simulink library "lib_lowphy"  (R2023b)
settings: Solver=VariableStepAuto  StartTime=0.0  StopTime=10.0  RelTol=1e-3
undefined symbols (not defined in the file or in its folder): AdvDSPBChannelOutDisplay, AdvDSPBDMemDisplay, AdvDSPBInDisplay, AdvDSPBOutDisplay, dpoly, dspba, dspba_ChannelInVis, dspba_ChannelOutVis, dspba_internal_get_channel_ports, evalAionMaskParam, fft_tb_in, ifft_tb_in, latency, latencyCorrection, max_FFTStages, max_NSubcarriers, primtype, UseDontCare, value
libraries: DSPBAPrim x637, DSPBAControl x55, $bdroot x16, DSPBAModelBus x12, DSPBAUtilities x6, DSPBABase x5, DSPBAWaveformSynth x4, DspbAdvFftLibrary x3, DSPBAVectorUtil x2, DspbAdvVfftPrefix x1
(part 4 of 9)

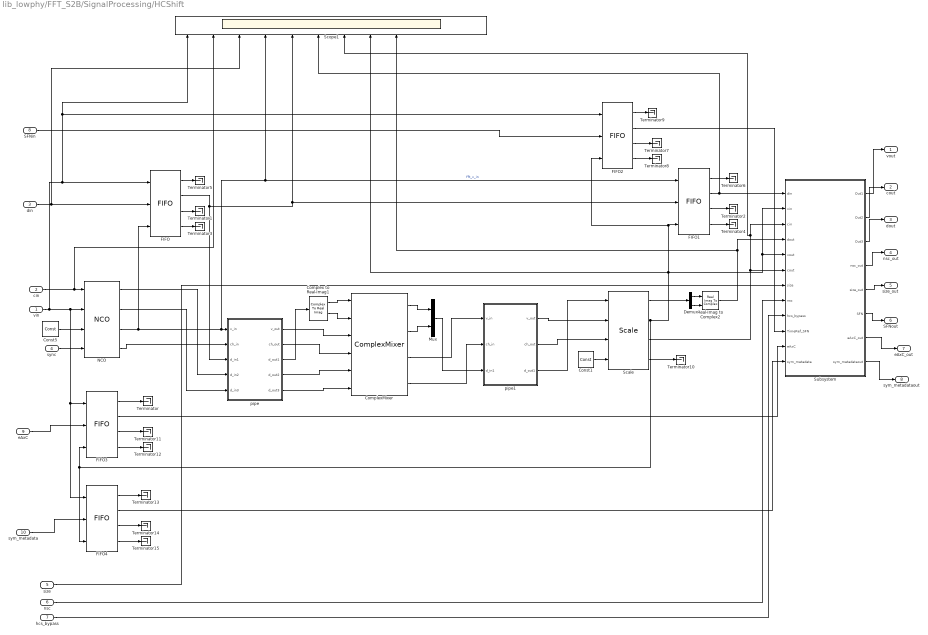
== system lib_lowphy/FFT_S2B/SignalProcessing/HCShift ==
  vin : Inport
  cin : Inport  Port=2
  din : Inport  Port=3
  sync : Inport  Port=4
  size : Inport  Port=5
  nsc : Inport  Port=6
  hcs_bypass : Inport  Port=7
  SFNin : Inport  Port=8
  eAxC : Inport  Port=9
  sym_metadata : Inport  Port=10
  Complex to Real-Imag1 : ComplexToRealImag
  ComplexMixer : DSPBAWaveformSynth/ComplexMixer  nInputRate=dspb_fft_multichannel.ClockRate  nchan=1  nfreq=1  latency=5  simulationMode=Use Global Value  version=20090407
  Const1 : DSPBAPrim/Const  primtype=const  nInputs=0  nOutputs=1  omode=Inherit via internal rule  otype=sfix(16)  scale=2^-15  rndmethod=Unbiased  factor=1  satmethod=Symmetric  shift_vec=[0 1 2 -1]  value=0  inPortNames=['+'; '+';]  outPortNames=[' ']  dspbaimage=dspba_prim.svg  text=fprintf('%s', num2str(value));  style=Optimised  visibilities=8 + 1024  floatPrecision=float32_m23  warnSaturation=on  version=20211007  SampleTime=inf
  Const5 : DSPBAPrim/Const  primtype=const  nInputs=0  nOutputs=1  omode=Specify via dialog  otype=uint(30)  scale=2^0  rndmethod=Unbiased  factor=1  satmethod=Symmetric  shift_vec=[0 1 2 -1]  value=0  inPortNames=['+'; '+';]  outPortNames=[' ']  dspbaimage=dspba_prim.svg  text=fprintf('%s', num2str(value));  style=Optimised  visibilities=8 + 1024  floatPrecision=float32_m23  warnSaturation=on  version=20211007  SampleTime=inf
  Demux : Demux  Outputs=2
  FIFO{,1,3..4} (4 alike) : DSPBAPrim/FIFO  primtype=fifo  nInputs=3  nOutputs=4  omode=Inherit via internal rule  otype=sfix(16)  scale=2^-15  rndmethod=Unbiased  factor=1  satmethod=Symmetric  shift_vec=[0 1 2 -1]  value=[32 4 16]  inPortNames=['w'; 'd'; 'r'; 'f']  outPortNames=['v'; 'q'; 't'; 'f']  dspbaimage=dspba_prim_tall.svg  text=fprintf('fifo');  style=Optimised  visibilities=263168  version=20211007  user_sclr=off
  FIFO2 : DSPBAPrim/FIFO  primtype=fifo  nInputs=3  nOutputs=4  omode=Inherit via internal rule  otype=sfix(16)  scale=2^-15  rndmethod=Unbiased  factor=1  satmethod=Symmetric  shift_vec=[0 1 2 -1]  value=[64 4 16]  inPortNames=['w'; 'd'; 'r'; 'f']  outPortNames=['v'; 'q'; 't'; 'f']  dspbaimage=dspba_prim_tall.svg  text=fprintf('fifo');  style=Optimised  visibilities=263168  version=20211007  user_sclr=off
  Mux : Mux  Inputs=2
  NCO : DSPBAWaveformSynth/NCO  outputRate=dspb_fft_multichannel.ClockRate  otype=sfix(18)  scale=2^-17  accumBitWidth=30  phaseIncrAndInv=7.5e3*2^30/7.68e6  phaseIncrAndInvMap=NCO_addr_offset  rwmode=Read/Write  exposebus=off  version=20090407  SampleTime=-1  expSFDR=108.36  accumPrecision=+/- 0.22888  phaseIncrInMHz=[0.48]  outWidth=3  tableSize=8  latency=17
  Real-Imag to Complex2 : RealImagToComplex
  Scale : DSPBABase/Scale  otype=sfix(16)  scale=2^-15  rndmethod=Biased  factor=1  satmethod=Symmetric  shift_vec=0  latency=3  simulationMode=Use Global Value  version=20130807
  Scope1 : Scope  NumInputPorts=12
  Subsystem : Subsystem
  Terminator{,1..15} (16 alike) : Terminator
  pipe : Subsystem
  pipe1 : Subsystem
  vout : Outport
  cout : Outport  Port=2
  dout : Outport  Port=3
  nsc_out : Outport  Port=4
  size_out : Outport  Port=5
  SFNout : Outport  Port=6
  eAxC_out : Outport  Port=7
  sym_metadataout : Outport  Port=8
  wires:
  NCO/3 -> FIFO/3, FIFO1/1, Scope1/4, pipe/1(v_in)  "fft_v_in"
  Const5/1 -> NCO/3
  cin/1 -> Scope1/2, NCO/1
  vin/1 -> FIFO2/1, Scope1/1, FIFO/1, FIFO4/1, FIFO3/1, NCO/2
  Subsystem/1(Out1) -> vout/1
  Subsystem/2(Out2) -> cout/1
  Subsystem/3(Out3) -> dout/1
  FIFO/3 -> Terminator1/1
  FIFO/4 -> Terminator3/1
  nsc/1 -> Subsystem/8(nsc)
  size/1 -> Subsystem/7(size)
  Subsystem/5(size_out) -> size_out/1
  Subsystem/4(nsc_out) -> nsc_out/1
  hcs_bypass/1 -> Subsystem/9(hcs_bypass)
  sync/1 -> NCO/4
  Real-Imag to Complex2/1 -> Scope1/9, Subsystem/4(dout)
  Scale/2 -> FIFO4/3, FIFO3/3, Scope1/8, Subsystem/2(vin), Subsystem/5(vout), FIFO2/3, FIFO1/3
  Scale/3 -> Scope1/7, Subsystem/3(cin), Subsystem/6(cout)
  FIFO/2 -> FIFO1/2, Scope1/5, pipe/3(d_in1)
  NCO/1 -> pipe/4(d_in2)
  pipe1/1(v_out) -> Scale/2
  NCO/4 -> pipe/2(ch_in)
  Complex to Real-Imag1/2 -> ComplexMixer/2
  pipe1/2(ch_out) -> Scale/3
  pipe/3(d_out1) -> Complex to Real-Imag1/1
  pipe/1(v_out) -> ComplexMixer/3
  Demux/1 -> Real-Imag to Complex2/1
  pipe1/3(d_out1) -> Scale/1
  ComplexMixer/4 -> pipe1/2(ch_in)
  pipe/5(d_out3) -> ComplexMixer/6
  Scale/4 -> Terminator10/1
  pipe/4(d_out2) -> ComplexMixer/5
  Const1/1 -> Scale/4
  ComplexMixer/1 -> Mux/1
  Scale/1 -> Demux/1
  Complex to Real-Imag1/1 -> ComplexMixer/1
  Demux/2 -> Real-Imag to Complex2/2
  pipe/2(ch_out) -> ComplexMixer/4
  ComplexMixer/3 -> pipe1/1(v_in)
  Mux/1 -> pipe1/3(d_in1)
  ComplexMixer/2 -> Mux/2
  NCO/2 -> pipe/5(d_in3)
  FIFO1/2 -> Scope1/6, Subsystem/1(din)
  FIFO1/4 -> Terminator4/1
  FIFO1/3 -> Terminator2/1
  FIFO/1 -> Terminator5/1
  FIFO1/1 -> Terminator6/1
  din/1 -> Scope1/3, FIFO/2
  SFNin/1 -> FIFO2/2
  FIFO2/3 -> Terminator7/1
  FIFO2/4 -> Terminator8/1
  FIFO2/1 -> Terminator9/1
  FIFO2/2 -> Subsystem/10(TimeRef_SFN)
  Subsystem/6(SFN) -> SFNout/1
  eAxC/1 -> FIFO3/2
  sym_metadata/1 -> FIFO4/2
  FIFO3/1 -> Terminator/1
  FIFO3/3 -> Terminator11/1
  FIFO3/4 -> Terminator12/1
  FIFO4/1 -> Terminator13/1
  FIFO4/3 -> Terminator14/1
  FIFO4/4 -> Terminator15/1
  Subsystem/7(eAxC_out) -> eAxC_out/1
  Subsystem/8(sym_metadataout) -> sym_metadataout/1
  FIFO3/2 -> Subsystem/11(eAxC)
  FIFO4/2 -> Subsystem/12(sym_metadata)

== system lib_lowphy/FFT_S2B/SignalProcessing/RXGainComp ==
  vin : Inport
  chin : Inport  Port=2
  din : Inport  Port=3
  nsc : Inport  Port=4
  size : Inport  Port=5
  fft_gain_re : Inport  Port=6
  fft_gain_im : Inport  Port=7
  time_in : Inport  Port=8
  eAxC : Inport  Port=9
  sym_metadata : Inport  Port=10
  Mult : DSPBAPrim/Mult  primtype=mult  nInputs=2  nOutputs=1  omode=Inherit via internal rule  otype=sfix(16)  scale=2^-15  rndmethod=Unbiased  factor=1  satmethod=Symmetric  shift_vec=[0 1 2 -1]  value=0  inPortNames=[' '; ' ';]  outPortNames=[' ']  dspbaimage=dspba_prim.svg  text=fprintf('X');  style=Optimised  visibilities=8+2^18+2^19  floatPrecision=float32_m23  floatRounding=correct  advOptions=[]  version=20211007
  Real-Imag to Complex : RealImagToComplex
  Scale1 : DSPBAPrim/Convert  primtype=convert  nInputs=1  nOutputs=1  omode=Specify via dialog  otype=sfix(16)  scale=2^-14  rndmethod=Biased  factor=1  satmethod=Symmetric  shift_vec=[0 1 2 -1]  value=round([0:255]/17)  inPortNames=[' '; ' ';]  outPortNames=[' '; 'c']  dspbaimage=dspba_prim_wide.svg  text=fprintf('convert');  style=Optimised  visibilities=8+64+256+2^17  clipdetect=off  floatPrecision=float32_m23  advOptions=[]  version=20211007
  SynthesisInfo : DSPBAPrim/SynthesisInfo  primtype=synthinfo  nInputs=0  nOutputs=0  omode=Inherit via internal rule  otype=sfix(16)  scale=2^-15  rndmethod=Truncate  factor=1  satmethod=Symmetric  shift_vec=[0 1 2 -1]  value=99  inPortNames=[' '; ' ';]  outPortNames=[' ']  dspbaimage=dspba_prim_ctrl.jpg  text=fprintf('Style=%s', style);  style=Scheduled  visibilities=2^17+2^18+2^19+2^20+2^21+2^22+2^23+2^24  constraintPair=None  constraintRelation=>  constraintLimit=2  modelRefSign=+  modelRef=''  showSchedule=off  simulationMode=Use Global Value  resetMinimization=Conditional - On for ChannelIn/Out only  version=20220106
  channel_RXG1_in : DSPBAPrim/ChannelIn  primtype=channelin  nInputs=dspba_internal_get_channel_ports(gcb)  nOutputs=dspba_internal_get_channel_ports(gcb)  omode=Inherit via internal rule  otype=sfix(16)  scale=2^-15  rndmethod=Unbiased  factor=1  satmethod=Symmetric  shift_vec=[0 1 2 -1]  value=8  inPortNames=['v'; 'c'; '0'; '1'; '2'; '3'; '4'; '5'; '6'; '7'; '8'; '9'; 'A'; 'B'; 'D'; 'E'; 'F'; 'G'; 'H'; 'I'; 'J'; 'K'; 'L'; 'M'; 'N'; 'O'; 'P'; 'Q'; 'R'; 'S'; 'T'; 'U'; 'W'; 'X'; 'Y'; 'Z']  outPortNames=['v'; 'c'; '0'; '1'; '2'; '3'; '4'; '5'; '6'; '7'; '8'; '9'; 'A'; 'B'; 'D'; 'E'; 'F'; 'G'; 'H'; 'I'; 'J'; 'K'; 'L'; 'M'; 'N'; 'O'; 'P'; 'Q'; 'R'; 'S'; 'T'; 'U'; 'W'; 'X'; 'Y'; 'Z']  dspbaimage=dspba_prim_channel_tall.svg  text=fprintf('In');  style=Optimised  dataSignals=8  foldingEnabled=off  channels=1  sampleRate=200  packetBeginPresent=off  packetBeginEnabled=off  visibilities=dspba_ChannelInVis(gcb)  latencyCorrection=0  scheduleOrigin=on  version=20211214
  channel_RXG1_out : DSPBAPrim/ChannelOut  primtype=channelout  nInputs=dspba_internal_get_channel_ports(gcb)  nOutputs=dspba_internal_get_channel_ports(gcb)  omode=Inherit via internal rule  otype=sfix(16)  scale=2^-15  rndmethod=Unbiased  factor=1  satmethod=Symmetric  shift_vec=[0 1 2 -1]  value=6  inPortNames=['v'; 'c'; '0'; '1'; '2'; '3'; '4'; '5'; '6'; '7'; '8'; '9'; 'A'; 'B'; 'D'; 'E'; 'F'; 'G'; 'H'; 'I'; 'J'; 'K'; 'L'; 'M'; 'N'; 'O'; 'P'; 'Q'; 'R'; 'S'; 'T'; 'U'; 'W'; 'X'; 'Y'; 'Z']  outPortNames=['v'; 'c'; '0'; '1'; '2'; '3'; '4'; '5'; '6'; '7'; '8'; '9'; 'A'; 'B'; 'D'; 'E'; 'F'; 'G'; 'H'; 'I'; 'J'; 'K'; 'L'; 'M'; 'N'; 'O'; 'P'; 'Q'; 'R'; 'S'; 'T'; 'U'; 'W'; 'X'; 'Y'; 'Z']  dspbaimage=dspba_prim_channel_tall.svg  text=fprintf('Out%s', AdvDSPBChannelOutDisplay(latency));  style=Optimised  dataSignals=6  foldingEnabled=off  channels=1  sampleRate=200  packetBeginPresent=off  packetBeginEnabled=off  visibilities=dspba_ChannelOutVis(gcb)  latency=8  latencyCorrection=0  version=20211214
  vout : Outport
  chout : Outport  Port=2
  dout : Outport  Port=3
  nsc_out : Outport  Port=4
  size_out : Outport  Port=5
  time_out : Outport  Port=6
  eAxC_out : Outport  Port=7
  sym_metadata_out : Outport  Port=8
  wires:
  Scale1/1 -> channel_RXG1_out/3
  Mult/1 -> Scale1/1
  channel_RXG1_out/1 -> vout/1
  channel_RXG1_out/2 -> chout/1
  channel_RXG1_in/1 -> channel_RXG1_out/1
  channel_RXG1_in/2 -> channel_RXG1_out/2
  channel_RXG1_out/3 -> dout/1
  channel_RXG1_in/3 -> Mult/1
  chin/1 -> channel_RXG1_in/2
  vin/1 -> channel_RXG1_in/1
  din/1 -> channel_RXG1_in/3
  channel_RXG1_out/4 -> size_out/1
  channel_RXG1_out/5 -> nsc_out/1
  channel_RXG1_in/4 -> channel_RXG1_out/4
  channel_RXG1_in/5 -> channel_RXG1_out/5
  size/1 -> channel_RXG1_in/4
  nsc/1 -> channel_RXG1_in/5
  fft_gain_re/1 -> channel_RXG1_in/6
  fft_gain_im/1 -> channel_RXG1_in/7
  channel_RXG1_in/7 -> Real-Imag to Complex/2
  time_in/1 -> channel_RXG1_in/8
  channel_RXG1_in/8 -> channel_RXG1_out/6
  channel_RXG1_out/6 -> time_out/1
  channel_RXG1_in/6 -> Real-Imag to Complex/1
  Real-Imag to Complex/1 -> Mult/2
  eAxC/1 -> channel_RXG1_in/9
  sym_metadata/1 -> channel_RXG1_in/10
  channel_RXG1_out/7 -> eAxC_out/1
  channel_RXG1_out/8 -> sym_metadata_out/1
  channel_RXG1_in/9 -> channel_RXG1_out/7
  channel_RXG1_in/10 -> channel_RXG1_out/8

== system lib_lowphy/FFT_S2B/SignalProcessing/RXScaling ==
  vin : Inport
  chin : Inport  Port=2
  size : Inport  Port=3
  din : Inport  Port=4
  nsc : Inport  Port=5
  fft_shift : Inport  Port=6
  time_in : Inport  Port=7
  eAxC : Inport  Port=8
  sym_metadata : Inport  Port=9
  Complex to Real-Imag : ComplexToRealImag
  Real-Imag to Complex : RealImagToComplex
  Scale1 : DSPBAPrim/Convert  primtype=convert  nInputs=1  nOutputs=1  omode=Specify via dialog  otype=sfix(16)  scale=Rx_scaling  rndmethod=Biased  factor=1  satmethod=Symmetric  shift_vec=[0 1 2 -1]  value=round([0:255]/17)  inPortNames=[' '; ' ';]  outPortNames=[' '; 'c']  dspbaimage=dspba_prim_wide.svg  text=fprintf('convert');  style=Optimised  visibilities=8+64+256+2^17  clipdetect=off  floatPrecision=float32_m23  advOptions=[]  version=20211007
  Scale2 : DSPBAPrim/Convert  primtype=convert  nInputs=1  nOutputs=1  omode=Specify via dialog  otype=sfix(16)  scale=Rx_scaling  rndmethod=Biased  factor=1  satmethod=Symmetric  shift_vec=[0 1 2 -1]  value=round([0:255]/17)  inPortNames=[' '; ' ';]  outPortNames=[' '; 'c']  dspbaimage=dspba_prim_wide.svg  text=fprintf('convert');  style=Optimised  visibilities=8+64+256+2^17  clipdetect=off  floatPrecision=float32_m23  advOptions=[]  version=20211007
  Scope : Scope  NumInputPorts=3
  Shift : DSPBAPrim/Shift  primtype=shift  nInputs=2  nOutputs=1  omode=Inherit via internal rule  otype=sfix(16)  scale=Rx_scaling  rndmethod=Unbiased  factor=1  satmethod=Symmetric  shift_vec=[0 1 2 -1]  value=0  inPortNames=['a'; 'b';]  outPortNames=[' ']  dspbaimage=dspba_prim.svg  text=fprintf('a >> b');  style=Optimised  visibilities=8  version=20211007
  Shift1 : DSPBAPrim/Shift  primtype=shift  nInputs=2  nOutputs=1  omode=Inherit via internal rule  otype=sfix(16)  scale=Rx_scaling  rndmethod=Unbiased  factor=1  satmethod=Symmetric  shift_vec=[0 1 2 -1]  value=0  inPortNames=['a'; 'b';]  outPortNames=[' ']  dspbaimage=dspba_prim.svg  text=fprintf('a >> b');  style=Optimised  visibilities=8  version=20211007
  SynthesisInfo : DSPBAPrim/SynthesisInfo  primtype=synthinfo  nInputs=0  nOutputs=0  omode=Inherit via internal rule  otype=sfix(16)  scale=2^-15  rndmethod=Truncate  factor=1  satmethod=Symmetric  shift_vec=[0 1 2 -1]  value=99  inPortNames=[' '; ' ';]  outPortNames=[' ']  dspbaimage=dspba_prim_ctrl.jpg  text=fprintf('Style=%s', style);  style=Scheduled  visibilities=2^17+2^18+2^19+2^20+2^21+2^22+2^23+2^24  constraintPair=None  constraintRelation=>  constraintLimit=2  modelRefSign=+  modelRef=''  showSchedule=off  simulationMode=Use Global Value  resetMinimization=Conditional - On for ChannelIn/Out only  version=20220106
  channel_RXS1_in : DSPBAPrim/ChannelIn  primtype=channelin  nInputs=dspba_internal_get_channel_ports(gcb)  nOutputs=dspba_internal_get_channel_ports(gcb)  omode=Inherit via internal rule  otype=sfix(16)  scale=2^-15  rndmethod=Unbiased  factor=1  satmethod=Symmetric  shift_vec=[0 1 2 -1]  value=8  inPortNames=['v'; 'c'; '0'; '1'; '2'; '3'; '4'; '5'; '6'; '7'; '8'; '9'; 'A'; 'B'; 'D'; 'E'; 'F'; 'G'; 'H'; 'I'; 'J'; 'K'; 'L'; 'M'; 'N'; 'O'; 'P'; 'Q'; 'R'; 'S'; 'T'; 'U'; 'W'; 'X'; 'Y'; 'Z']  outPortNames=['v'; 'c'; '0'; '1'; '2'; '3'; '4'; '5'; '6'; '7'; '8'; '9'; 'A'; 'B'; 'D'; 'E'; 'F'; 'G'; 'H'; 'I'; 'J'; 'K'; 'L'; 'M'; 'N'; 'O'; 'P'; 'Q'; 'R'; 'S'; 'T'; 'U'; 'W'; 'X'; 'Y'; 'Z']  dspbaimage=dspba_prim_channel_tall.svg  text=fprintf('In');  style=Optimised  dataSignals=8  foldingEnabled=off  channels=1  sampleRate=200  packetBeginPresent=off  packetBeginEnabled=off  visibilities=dspba_ChannelInVis(gcb)  latencyCorrection=0  scheduleOrigin=on  version=20211214
  channel_RXS1_out : DSPBAPrim/ChannelOut  primtype=channelout  nInputs=dspba_internal_get_channel_ports(gcb)  nOutputs=dspba_internal_get_channel_ports(gcb)  omode=Inherit via internal rule  otype=sfix(16)  scale=2^-15  rndmethod=Unbiased  factor=1  satmethod=Symmetric  shift_vec=[0 1 2 -1]  value=7  inPortNames=['v'; 'c'; '0'; '1'; '2'; '3'; '4'; '5'; '6'; '7'; '8'; '9'; 'A'; 'B'; 'D'; 'E'; 'F'; 'G'; 'H'; 'I'; 'J'; 'K'; 'L'; 'M'; 'N'; 'O'; 'P'; 'Q'; 'R'; 'S'; 'T'; 'U'; 'W'; 'X'; 'Y'; 'Z']  outPortNames=['v'; 'c'; '0'; '1'; '2'; '3'; '4'; '5'; '6'; '7'; '8'; '9'; 'A'; 'B'; 'D'; 'E'; 'F'; 'G'; 'H'; 'I'; 'J'; 'K'; 'L'; 'M'; 'N'; 'O'; 'P'; 'Q'; 'R'; 'S'; 'T'; 'U'; 'W'; 'X'; 'Y'; 'Z']  dspbaimage=dspba_prim_channel_tall.svg  text=fprintf('Out%s', AdvDSPBChannelOutDisplay(latency));  style=Optimised  dataSignals=7  foldingEnabled=off  channels=1  sampleRate=200  packetBeginPresent=off  packetBeginEnabled=off  visibilities=dspba_ChannelOutVis(gcb)  latency=6  latencyCorrection=0  version=20211214
  vout : Outport
  chout : Outport  Port=2
  dout : Outport  Port=3
  size_out : Outport  Port=4
  nsc_out : Outport  Port=5
  time_out : Outport  Port=6
  eAxCout : Outport  Port=7
  sym_metadataout : Outport  Port=8
  wires:
  channel_RXS1_out/7 -> time_out/1
  channel_RXS1_out/6 -> nsc_out/1
  channel_RXS1_out/2 -> chout/1
  Scale1/1 -> channel_RXS1_out/3
  Shift/1 -> Scale1/1
  channel_RXS1_in/8 -> channel_RXS1_out/7
  channel_RXS1_in/7 -> Shift/2, Shift1/2
  channel_RXS1_in/6 -> channel_RXS1_out/6
  channel_RXS1_in/5 -> channel_RXS1_out/5
  channel_RXS1_out/1 -> vout/1
  nsc/1 -> channel_RXS1_in/6
  din/1 -> Complex to Real-Imag/1
  size/1 -> channel_RXS1_in/5
  channel_RXS1_out/5 -> size_out/1
  vin/1 -> channel_RXS1_in/1
  channel_RXS1_in/2 -> channel_RXS1_out/2
  Complex to Real-Imag/1 -> channel_RXS1_in/3
  fft_shift/1 -> channel_RXS1_in/7
  chin/1 -> channel_RXS1_in/2
  time_in/1 -> channel_RXS1_in/8
  Complex to Real-Imag/2 -> channel_RXS1_in/4
  channel_RXS1_in/1 -> channel_RXS1_out/1
  Real-Imag to Complex/1 -> dout/1
  channel_RXS1_out/4 -> Real-Imag to Complex/2
  channel_RXS1_out/3 -> Real-Imag to Complex/1
  Shift1/1 -> Scale2/1
  channel_RXS1_in/3 -> Scope/1, Shift/1, Scope/2
  Scale2/1 -> channel_RXS1_out/4
  channel_RXS1_in/4 -> Shift1/1
  eAxC/1 -> channel_RXS1_in/9
  sym_metadata/1 -> channel_RXS1_in/10
  channel_RXS1_out/8 -> eAxCout/1
  channel_RXS1_out/9 -> sym_metadataout/1
  channel_RXS1_in/9 -> channel_RXS1_out/8
  channel_RXS1_in/10 -> channel_RXS1_out/9

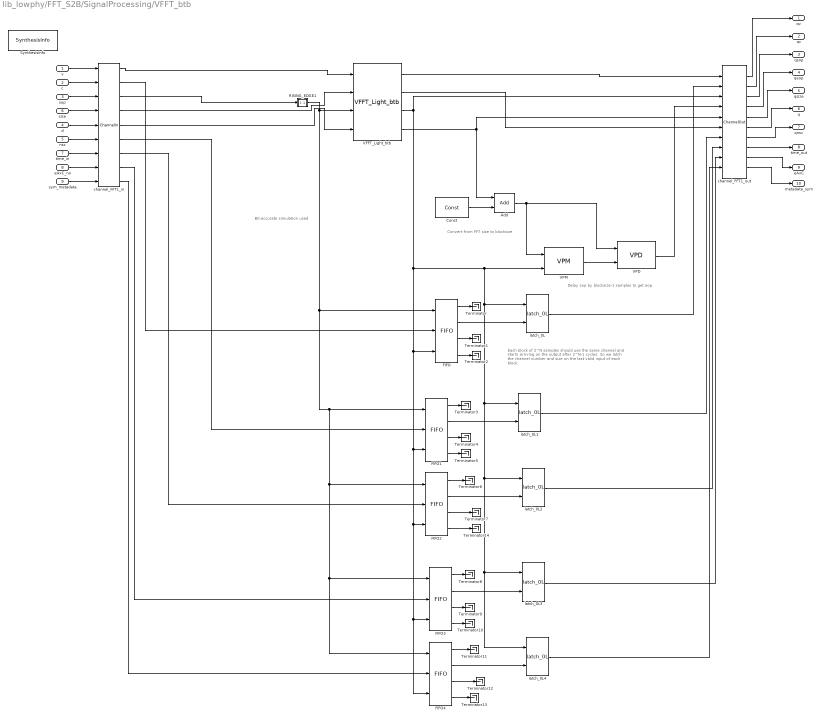
== system lib_lowphy/FFT_S2B/SignalProcessing/VFFT_btb ==
  note: Bit-accurate simulation used
  note: Each block of 2^N samples should use the same channel
      | and starts arriving on the output after 2^N-1 cycles.
      |
      | So we latch the channel number and size on
      |  the last valid input of each block.
  note: Convert from FFT size to blocksize
  note: Delay sop by blocksize-1 samples to get eop.
  v : Inport
  c : Inport  Port=2
  sop : Inport  Port=3
  d : Inport  Port=4
  nsc : Inport  Port=5
  size : Inport  Port=6
  time_in : Inport  Port=7
  eAxC_no : Inport  Port=8
  sym_metadata : Inport  Port=9
  Add : DSPBAPrim/Add  primtype=add  nInputs=evalAionMaskParam(gcb,'value',1)  nOutputs=1  omode=Specify via dialog  otype=fixdt(0,adderWidth,0)  scale=0  rndmethod=Unbiased  factor=1  satmethod=Symmetric  shift_vec=[0 1 2 -1]  value=2  inPortNames=[' '; ' ';]  outPortNames=[' ']  dspbaimage=dspba_prim.svg  text=fprintf('+');  style=Optimised  visibilities=1032+2^17+2^18+2^19  genFPC=off  floatRounding=correct  advOptions=[]  version=20211007
  Const : DSPBAPrim/Const  primtype=const  nInputs=0  nOutputs=1  omode=Inherit via internal rule  otype=sfix(16)  scale=2^-15  rndmethod=Unbiased  factor=1  satmethod=Symmetric  shift_vec=[0 1 2 -1]  value=subchannelbits  inPortNames=['+'; '+';]  outPortNames=[' ']  dspbaimage=dspba_prim.svg  text=fprintf('%s', num2str(value));  style=Optimised  visibilities=8 + 1024  floatPrecision=float32_m23  warnSaturation=on  version=20211007  SampleTime=inf
  FIFO{,1..4} (5 alike) : DSPBAPrim/FIFO  primtype=fifo  nInputs=3  nOutputs=4  omode=Inherit via internal rule  otype=sfix(16)  scale=2^-15  rndmethod=Unbiased  factor=1  satmethod=Symmetric  shift_vec=[0 1 2 -1]  value=[2^(maxSize-minSize) 4 16]  inPortNames=['w'; 'd'; 'r'; 'f']  outPortNames=['v'; 'q'; 't'; 'f']  dspbaimage=dspba_prim_tall.svg  text=fprintf('fifo');  style=Optimised  visibilities=263168  version=20211007  user_sclr=off
  RISING_EDGE1 : Subsystem
  SynthesisInfo : DSPBAPrim/SynthesisInfo  primtype=synthinfo  nInputs=0  nOutputs=0  omode=Inherit via internal rule  otype=sfix(16)  scale=2^-15  rndmethod=Truncate  factor=1  satmethod=Symmetric  shift_vec=[0 1 2 -1]  value=99  inPortNames=[' '; ' ';]  outPortNames=[' ']  dspbaimage=dspba_prim_ctrl.jpg  text=fprintf('Style=%s', style);  style=Scheduled  visibilities=2^17+2^18+2^19+2^20+2^21+2^22+2^23+2^24  constraintPair=None  constraintRelation=>  constraintLimit=2  modelRefSign=+  modelRef=''  showSchedule=off  simulationMode=Bit Accurate  resetMinimization=Conditional - On for ChannelIn/Out only  version=20220106
  Terminator{,1..14} (15 alike) : Terminator
  VFFT_Light_btb : DspbAdvVfftPrefix/VFFT_Light_btb  IFFT=IFFT  subchannels=subchannels  br_in=br_in  maxSize=maxSize  minSize=minSize  in_type=in_type  type_strings=type_strings  faithful=faithful  wirecount=1
  VPD : DspbAdvFftLibrary/Private/VPD  N=maxBlocksizeBits
  VPM : DspbAdvFftLibrary/Private/VPM  N=maxBlocksizeBits
  channel_FFT1_in : DSPBAPrim/ChannelIn  primtype=channelin  nInputs=dspba_internal_get_channel_ports(gcb)  nOutputs=dspba_internal_get_channel_ports(gcb)  omode=Inherit via internal rule  otype=sfix(16)  scale=2^-15  rndmethod=Unbiased  factor=1  satmethod=Symmetric  shift_vec=[0 1 2 -1]  value=7  inPortNames=['v'; 'c'; '0'; '1'; '2'; '3'; '4'; '5'; '6'; '7'; '8'; '9'; 'a'; 'b']  outPortNames=['v'; 'c'; '0'; '1'; '2'; '3'; '4'; '5'; '6'; '7'; '8'; '9'; 'a'; 'b']  dspbaimage=dspba_prim_channel_tall.svg  text=fprintf('In');  style=Optimised  dataSignals=7  foldingEnabled=off  channels=1  sampleRate=200  packetBeginPresent=off  packetBeginEnabled=off  visibilities=dspba_ChannelInVis(gcb)  latencyCorrection=0  scheduleOrigin=on  version=20211214
  channel_FFT1_out : DSPBAPrim/ChannelOut  primtype=channelout  nInputs=dspba_internal_get_channel_ports(gcb)  nOutputs=dspba_internal_get_channel_ports(gcb)  omode=Inherit via internal rule  otype=sfix(16)  scale=2^-15  rndmethod=Unbiased  factor=1  satmethod=Symmetric  shift_vec=[0 1 2 -1]  value=8  inPortNames=['v'; 'c'; '0'; '1'; '2'; '3'; '4'; '5'; '6'; '7'; '8'; '9']  outPortNames=['v'; 'c'; '0'; '1'; '2'; '3'; '4'; '5'; '6'; '7'; '8'; '9']  dspbaimage=dspba_prim_channel_tall.svg  text=fprintf('Out');  style=Optimised  dataSignals=8  foldingEnabled=off  channels=1  sampleRate=200  packetBeginPresent=off  packetBeginEnabled=off  visibilities=dspba_ChannelOutVis(gcb)  latency=75  latencyCorrection=0  version=20211214
  latch_0L{,1..4} (5 alike) : DSPBAControl/latch_0L
  qv : Outport
  qc : Outport  Port=2
  qsop : Outport  Port=3
  qeop : Outport  Port=4
  qsize : Outport  Port=5
  q : Outport  Port=6
  qnsc : Outport  Port=7
  time_out : Outport  Port=8
  eAxC : Outport  Port=9
  metadata_sym : Outport  Port=10
  wires:
  v/1 -> channel_FFT1_in/1
  c/1 -> channel_FFT1_in/2
  channel_FFT1_out/1 -> qv/1
  channel_FFT1_out/2 -> qc/1
  VFFT_Light_btb/1 -> channel_FFT1_out/1
  sop/1 -> channel_FFT1_in/3
  channel_FFT1_out/3 -> qsop/1
  size/1 -> channel_FFT1_in/4
  d/1 -> channel_FFT1_in/5
  channel_FFT1_in/1 -> VFFT_Light_btb/1
  channel_FFT1_in/2 -> FIFO/2
  RISING_EDGE1/1(q) -> FIFO/1, FIFO4/1, FIFO3/1, FIFO2/1, FIFO1/1, VFFT_Light_btb/3
  FIFO/2 -> latch_0L/2
  latch_0L/1 -> channel_FFT1_out/2
  FIFO/1 -> Terminator/1
  FIFO/3 -> Terminator1/1
  FIFO/4 -> Terminator2/1
  channel_FFT1_in/4 -> VFFT_Light_btb/2
  channel_FFT1_in/5 -> VFFT_Light_btb/4
  VPM/1 -> VPD/2
  channel_FFT1_out/6 -> q/1
  channel_FFT1_out/5 -> qsize/1
  channel_FFT1_out/4 -> qeop/1
  VFFT_Light_btb/2 -> channel_FFT1_out/6
  VPD/1 -> channel_FFT1_out/4
  VFFT_Light_btb/4 -> Add/1, channel_FFT1_out/5
  Add/1 -> VPD/1, VPM/1
  Const/1 -> Add/2
  nsc/1 -> channel_FFT1_in/6
  latch_0L1/1 -> channel_FFT1_out/7
  channel_FFT1_out/7 -> qnsc/1
  FIFO1/4 -> Terminator5/1
  FIFO1/3 -> Terminator4/1
  FIFO1/1 -> Terminator3/1
  FIFO1/2 -> latch_0L1/2
  channel_FFT1_in/6 -> FIFO1/2
  channel_FFT1_in/3 -> RISING_EDGE1/1(d)
  time_in/1 -> channel_FFT1_in/7
  channel_FFT1_out/8 -> time_out/1
  VFFT_Light_btb/3 -> channel_FFT1_out/3, FIFO4/3, FIFO3/3, FIFO2/3, FIFO1/3, FIFO/3, latch_0L4/1, latch_0L3/1, latch_0L2/1, latch_0L1/1, latch_0L/1, VPM/2
  FIFO2/1 -> Terminator6/1
  FIFO2/2 -> latch_0L2/2
  latch_0L2/1 -> channel_FFT1_out/8
  FIFO2/3 -> Terminator7/1
  channel_FFT1_in/7 -> FIFO2/2
  eAxC_no/1 -> channel_FFT1_in/8
  sym_metadata/1 -> channel_FFT1_in/9
  FIFO3/4 -> Terminator10/1
  FIFO3/1 -> Terminator8/1
  FIFO3/2 -> latch_0L3/2
  FIFO4/2 -> latch_0L4/2
  FIFO4/3 -> Terminator12/1
  FIFO3/3 -> Terminator9/1
  FIFO4/1 -> Terminator11/1
  FIFO4/4 -> Terminator13/1
  channel_FFT1_out/9 -> eAxC/1
  channel_FFT1_out/10 -> metadata_sym/1
  channel_FFT1_in/8 -> FIFO3/2
  channel_FFT1_in/9 -> FIFO4/2
  latch_0L3/1 -> channel_FFT1_out/9
  latch_0L4/1 -> channel_FFT1_out/10
  FIFO2/4 -> Terminator14/1

== system lib_lowphy/PhaseCompensation/PhasorGenerate/ChangeDetection ==
  In1 : Inport
  CmpNE : DSPBAPrim/CmpNE  primtype=cmpne  nInputs=2  nOutputs=1  omode=boolean  otype=sfix(16)  scale=2^-15  rndmethod=Unbiased  factor=1  satmethod=Symmetric  shift_vec=[0 1 2 -1]  value=0  inPortNames=[' '; ' ';]  outPortNames=[' ']  dspbaimage=dspba_prim.svg  text=fprintf('~=');  style=Optimised  visibilities=0  advOptions=[]  version=20211007
  SampleDelay : DSPBAPrim/SampleDelay  primtype=sampdelay  nInputs=1  nOutputs=1  omode=Inherit via internal rule  otype=sfix(16)  scale=2^-15  rndmethod=Unbiased  factor=1  satmethod=Symmetric  shift_vec=[0 1 2 -1]  floatPrecision=float32_m23  value=1  inPortNames=[' '; ' ';]  outPortNames=[' ']  dspbaimage=dspba_prim.svg  text=dpoly(1, eye(1,value+1), 'z')  style=Optimised  visibilities=8 + 1024 + 2^17 + 2^18  flexible=off  slackgroup=0  augmented=0  version=20211007  advOptions=[]
  Out1 : Outport
  wires:
  In1/1 -> CmpNE/1, SampleDelay/1
  SampleDelay/1 -> CmpNE/2
  CmpNE/1 -> Out1/1

== system lib_lowphy/PhaseCompensation_lite/SOP_EOP_gen/Rising_edge ==
  in : Inport
  Const : DSPBAPrim/Const  primtype=const  nInputs=0  nOutputs=1  omode=Specify via dialog  otype=ufix(1)  scale=0  rndmethod=Unbiased  factor=1  satmethod=Symmetric  shift_vec=[0 1 2 -1]  value=1  inPortNames=['+'; '+';]  outPortNames=[' ']  dspbaimage=dspba_prim.svg  text=fprintf('%s', num2str(value));  style=Optimised  visibilities=8 + 1024 + 2^18 + 2^20  floatPrecision=float32_m23  warnSaturation=on  version=20211007  SampleTime=inf
  Convert : DSPBAPrim/Convert  primtype=convert  nInputs=1  nOutputs=1  omode=Specify via dialog  otype=ufix(1)  scale=0  rndmethod=Unbiased  factor=1  satmethod=None  shift_vec=[0 1 2 -1]  value=round([0:255]/17)  inPortNames=[' '; ' ';]  outPortNames=[' '; 'c']  dspbaimage=dspba_prim_wide.svg  text=fprintf('convert');  style=Optimised  visibilities=8+64+256+2^17  clipdetect=off  floatPrecision=float32_m23  advOptions=[]  version=20211007
  Finite State Machine : DSPBAUtilities/Finite State Machine  desc_file=fsm_control_rising_edge.fsm  latency=0  simulationMode=Bit And Cycle Accurate  finiteStateMachine=on
  GPIn : DSPBAPrim/GPIn  Commented=through  primtype=gpin  nInputs=evalAionMaskParam(gcb,'value',1)  nOutputs=evalAionMaskParam(gcb,'value',1)  omode=Inherit via internal rule  otype=sfix(16)  scale=2^-15  rndmethod=Unbiased  factor=1  satmethod=Symmetric  shift_vec=[0 1 2 -1]  value=1  inPortNames=[' ' ' ' ' ' ' ' ' ' ' ' ' ' ' ' ' ' ' ' ' ' ' ' ' ' ' ' ' ' ' ' ' ' ' ' ' ' ' ' ' ' ' ' ' ' ' ' ' ' ' ' ' ' ' ' ' ' ' ' ' ' ' ' ' ' ' ' ' ']'  outPortNames=[' ' ' ' ' ' ' ' ' ' ' ' ' ' ' ' ' ' ' ' ' ' ' ' ' ' ' ' ' ' ' ' ' ' ' ' ' ' ' ' ' ' ' ' ' ' ' ' ' ' ' ' ' ' ' ' ' ' ' ' ' ' ' ' ' ' ' ' ' ']'  dspbaimage=dspba_prim_channel_tall.svg  text=fprintf('GPIn%s', AdvDSPBInDisplay(latencyCorrection));  style=Optimised  visibilities=1024  latencyCorrection=0  scheduleOrigin=on  version=20211214
  GPOut : DSPBAPrim/GPOut  Commented=through  primtype=gpout  nInputs=evalAionMaskParam(gcb,'value',1)  nOutputs=evalAionMaskParam(gcb,'value',1)  omode=Inherit via internal rule  otype=sfix(16)  scale=2^-15  rndmethod=Unbiased  factor=1  satmethod=Symmetric  shift_vec=[0 1 2 -1]  value=1  inPortNames=[' ' ' ' ' ' ' ' ' ' ' ' ' ' ' ' ' ' ' ' ' ' ' ' ' ' ' ' ' ' ' ' ' ' ' ' ' ' ' ' ' ' ' ' ' ' ' ' ' ' ' ' ' ' ' ' ' ' ' ' ' ' ' ' ' ' ' ' ' ']'  outPortNames=[' ' ' ' ' ' ' ' ' ' ' ' ' ' ' ' ' ' ' ' ' ' ' ' ' ' ' ' ' ' ' ' ' ' ' ' ' ' ' ' ' ' ' ' ' ' ' ' ' ' ' ' ' ' ' ' ' ' ' ' ' ' ' ' ' ' ' ' ' ']'  dspbaimage=dspba_prim_channel_tall.svg  text=fprintf('GPOut%s', AdvDSPBOutDisplay(latency, latencyCorrection));  style=Optimised  visibilities=1024  latency=0  latencyCorrection=0  version=20211214
  SynthesisInfo : DSPBAPrim/SynthesisInfo  Commented=on  primtype=synthinfo  nInputs=0  nOutputs=0  omode=Inherit via internal rule  otype=sfix(16)  scale=2^-15  rndmethod=Truncate  factor=1  satmethod=Symmetric  shift_vec=[0 1 2 -1]  value=99  inPortNames=[' '; ' ';]  outPortNames=[' ']  dspbaimage=dspba_prim_ctrl.jpg  text=fprintf('Style=%s', style);  style=Scheduled  visibilities=2^17+2^18+2^19+2^20+2^21+2^22+2^23+2^24  constraintPair=GPIn to GPOut  constraintRelation==  constraintLimit=0  modelRefSign=+  modelRef=''  showSchedule=off  simulationMode=Use Global Value  resetMinimization=Conditional - On for ChannelIn/Out only  version=20220106
  rising_edge : Outport
  wires:
  Convert/1 -> Finite State Machine/2
  in/1 -> GPIn/1
  GPOut/1 -> rising_edge/1
  Const/1 -> Finite State Machine/1
  Finite State Machine/1 -> GPOut/1
  GPIn/1 -> Convert/1

== system lib_lowphy/PhaseCompensation_lite/SOP_EOP_gen/falling_edge ==
  in : Inport
  Const : DSPBAPrim/Const  primtype=const  nInputs=0  nOutputs=1  omode=Specify via dialog  otype=ufix(1)  scale=0  rndmethod=Unbiased  factor=1  satmethod=Symmetric  shift_vec=[0 1 2 -1]  value=1  inPortNames=['+'; '+';]  outPortNames=[' ']  dspbaimage=dspba_prim.svg  text=fprintf('%s', num2str(value));  style=Optimised  visibilities=8 + 1024 + 2^18 + 2^20  floatPrecision=float32_m23  warnSaturation=on  version=20211007  SampleTime=inf
  Convert : DSPBAPrim/Convert  primtype=convert  nInputs=1  nOutputs=1  omode=Specify via dialog  otype=ufix(1)  scale=0  rndmethod=Unbiased  factor=1  satmethod=None  shift_vec=[0 1 2 -1]  value=round([0:255]/17)  inPortNames=[' '; ' ';]  outPortNames=[' '; 'c']  dspbaimage=dspba_prim_wide.svg  text=fprintf('convert');  style=Optimised  visibilities=8+64+256+2^17  clipdetect=off  floatPrecision=float32_m23  advOptions=[]  version=20211007
  Finite State Machine : DSPBAUtilities/Finite State Machine  desc_file=fsm_control_falling_edge.fsm  latency=0  simulationMode=Bit And Cycle Accurate  finiteStateMachine=on
  GPIn : DSPBAPrim/GPIn  Commented=through  primtype=gpin  nInputs=evalAionMaskParam(gcb,'value',1)  nOutputs=evalAionMaskParam(gcb,'value',1)  omode=Inherit via internal rule  otype=sfix(16)  scale=2^-15  rndmethod=Unbiased  factor=1  satmethod=Symmetric  shift_vec=[0 1 2 -1]  value=1  inPortNames=[' ' ' ' ' ' ' ' ' ' ' ' ' ' ' ' ' ' ' ' ' ' ' ' ' ' ' ' ' ' ' ' ' ' ' ' ' ' ' ' ' ' ' ' ' ' ' ' ' ' ' ' ' ' ' ' ' ' ' ' ' ' ' ' ' ' ' ' ' ']'  outPortNames=[' ' ' ' ' ' ' ' ' ' ' ' ' ' ' ' ' ' ' ' ' ' ' ' ' ' ' ' ' ' ' ' ' ' ' ' ' ' ' ' ' ' ' ' ' ' ' ' ' ' ' ' ' ' ' ' ' ' ' ' ' ' ' ' ' ' ' ' ' ']'  dspbaimage=dspba_prim_channel_tall.svg  text=fprintf('GPIn%s', AdvDSPBInDisplay(latencyCorrection));  style=Optimised  visibilities=1024  latencyCorrection=0  scheduleOrigin=on  version=20211214
  GPOut : DSPBAPrim/GPOut  Commented=through  primtype=gpout  nInputs=evalAionMaskParam(gcb,'value',1)  nOutputs=evalAionMaskParam(gcb,'value',1)  omode=Inherit via internal rule  otype=sfix(16)  scale=2^-15  rndmethod=Unbiased  factor=1  satmethod=Symmetric  shift_vec=[0 1 2 -1]  value=1  inPortNames=[' ' ' ' ' ' ' ' ' ' ' ' ' ' ' ' ' ' ' ' ' ' ' ' ' ' ' ' ' ' ' ' ' ' ' ' ' ' ' ' ' ' ' ' ' ' ' ' ' ' ' ' ' ' ' ' ' ' ' ' ' ' ' ' ' ' ' ' ' ']'  outPortNames=[' ' ' ' ' ' ' ' ' ' ' ' ' ' ' ' ' ' ' ' ' ' ' ' ' ' ' ' ' ' ' ' ' ' ' ' ' ' ' ' ' ' ' ' ' ' ' ' ' ' ' ' ' ' ' ' ' ' ' ' ' ' ' ' ' ' ' ' ' ']'  dspbaimage=dspba_prim_channel_tall.svg  text=fprintf('GPOut%s', AdvDSPBOutDisplay(latency, latencyCorrection));  style=Optimised  visibilities=1024  latency=0  latencyCorrection=0  version=20211214
  SynthesisInfo : DSPBAPrim/SynthesisInfo  Commented=on  primtype=synthinfo  nInputs=0  nOutputs=0  omode=Inherit via internal rule  otype=sfix(16)  scale=2^-15  rndmethod=Truncate  factor=1  satmethod=Symmetric  shift_vec=[0 1 2 -1]  value=99  inPortNames=[' '; ' ';]  outPortNames=[' ']  dspbaimage=dspba_prim_ctrl.jpg  text=fprintf('Style=%s', style);  style=Scheduled  visibilities=2^17+2^18+2^19+2^20+2^21+2^22+2^23+2^24  constraintPair=GPIn to GPOut  constraintRelation==  constraintLimit=0  modelRefSign=+  modelRef=''  showSchedule=off  simulationMode=Use Global Value  resetMinimization=Conditional - On for ChannelIn/Out only  version=20220106
  falling_edge : Outport
  wires:
  Convert/1 -> Finite State Machine/2
  in/1 -> GPIn/1
  GPOut/1 -> falling_edge/1
  Const/1 -> Finite State Machine/1
  Finite State Machine/1 -> GPOut/1
  GPIn/1 -> Convert/1

== system lib_lowphy/iFFT_B2S/B2S/B2S_Inst ==
  vin : Inport
  chin : Inport  Port=2
  din : Inport  Port=3
  FFTSize : Inport  Port=4
  cplen : Inport  Port=5
  nprb : Inport  Port=6
  BitCombine : DSPBAPrim/BitCombine  primtype=bitcombine  nInputs=2  nOutputs=1  omode=Inherit via internal rule  otype=sfix(16)  scale=2^-15  rndmethod=Unbiased  factor=1  satmethod=Symmetric  shift_vec=[0 1 2 -1]  value=0  inPortNames=['l'; 'h';]  outPortNames=[' ']  dspbaimage=dspba_prim.svg  text=fprintf('[h,l]');  style=Optimised  visibilities=8+2  version=20211007
  CB : Subsystem
  GPIn : DSPBAPrim/GPIn  primtype=gpin  nInputs=evalAionMaskParam(gcb,'value',1)  nOutputs=evalAionMaskParam(gcb,'value',1)  omode=Inherit via internal rule  otype=sfix(16)  scale=2^-15  rndmethod=Unbiased  factor=1  satmethod=Symmetric  shift_vec=[0 1 2 -1]  value=6  inPortNames=[' ' ' ' ' ' ' ' ' ' ' ' ' ' ' ' ' ' ' ' ' ' ' ' ' ' ' ' ' ' ' ' ' ' ' ' ' ' ' ' ' ' ' ' ' ' ' ' ' ' ' ' ' ' ' ' ' ' ' ' ' ' ' ' ' ' ' ' ' ']'  outPortNames=[' ' ' ' ' ' ' ' ' ' ' ' ' ' ' ' ' ' ' ' ' ' ' ' ' ' ' ' ' ' ' ' ' ' ' ' ' ' ' ' ' ' ' ' ' ' ' ' ' ' ' ' ' ' ' ' ' ' ' ' ' ' ' ' ' ' ' ' ' ']'  dspbaimage=dspba_prim_channel_tall.svg  text=fprintf('GPIn');  style=Optimised  visibilities=1024  latencyCorrection=0  scheduleOrigin=on  version=20211214
  GPOut : DSPBAPrim/GPOut  primtype=gpout  nInputs=evalAionMaskParam(gcb,'value',1)  nOutputs=evalAionMaskParam(gcb,'value',1)  omode=Inherit via internal rule  otype=sfix(16)  scale=2^-15  rndmethod=Unbiased  factor=1  satmethod=Symmetric  shift_vec=[0 1 2 -1]  value=3  inPortNames=[' ' ' ' ' ' ' ' ' ' ' ' ' ' ' ' ' ' ' ' ' ' ' ' ' ' ' ' ' ' ' ' ' ' ' ' ' ' ' ' ' ' ' ' ' ' ' ' ' ' ' ' ' ' ' ' ' ' ' ' ' ' ' ' ' ' ' ' ' ']'  outPortNames=[' ' ' ' ' ' ' ' ' ' ' ' ' ' ' ' ' ' ' ' ' ' ' ' ' ' ' ' ' ' ' ' ' ' ' ' ' ' ' ' ' ' ' ' ' ' ' ' ' ' ' ' ' ' ' ' ' ' ' ' ' ' ' ' ' ' ' ' ' ']'  dspbaimage=dspba_prim_channel_tall.svg  text=fprintf('GPOut');  style=Optimised  visibilities=1024  latency=8  latencyCorrection=0  version=20211214
  MemandMux : Subsystem
  SynthesisInfo : DSPBAPrim/SynthesisInfo  primtype=synthinfo  nInputs=0  nOutputs=0  omode=Inherit via internal rule  otype=sfix(16)  scale=2^-15  rndmethod=Truncate  factor=1  satmethod=Symmetric  shift_vec=[0 1 2 -1]  value=99  inPortNames=[' '; ' ';]  outPortNames=[' ']  dspbaimage=dspba_prim_ctrl.jpg  text=fprintf('Style=%s', style);  style=Scheduled  visibilities=2^17+2^18+2^19+2^20+2^21+2^22+2^23+2^24  constraintPair=GPIn to GPOut  constraintRelation=>=  constraintLimit=2  modelRefSign=+  modelRef=''  showSchedule=off  simulationMode=Use Global Value  resetMinimization=On - Always (for ChannelIn/Out or GPIn/Out)  version=20220106
  vout : Outport  VectorParamsAs1DForOutWhenUnconnected=off
  cout : Outport  Port=2  VectorParamsAs1DForOutWhenUnconnected=off
  q : Outport  Port=3  VectorParamsAs1DForOutWhenUnconnected=off
  wires:
  GPIn/5 -> CB/4(cplen)
  CB/7(AntNo) -> MemandMux/4(Ant_sel)
  GPIn/1 -> CB/1(vin)
  GPIn/2 -> CB/2(chin)
  GPIn/3 -> MemandMux/5(data_in)  "data_in"
  GPIn/4 -> CB/3(FFTSize)
  CB/5(rba) -> BitCombine/2
  CB/8(rdaddr1) -> BitCombine/1
  CB/2(Wr_Antenna_no) -> MemandMux/2(AntennaCurId)
  CB/3(Wr_ptr) -> MemandMux/3(Wraddr)
  BitCombine/1 -> MemandMux/6(rdaddr)
  MemandMux/1(dout) -> GPOut/1
  MemandMux/3(dv_out) -> GPOut/3
  MemandMux/2(ch_out) -> GPOut/2
  CB/1(rddv) -> MemandMux/7(rd_dv_in)
  CB/6(We) -> MemandMux/1(dv_we)
  vin/1 -> GPIn/1
  chin/1 -> GPIn/2
  din/1 -> GPIn/3  "data_in"
  FFTSize/1 -> GPIn/4
  cplen/1 -> GPIn/5
  GPOut/2 -> cout/1
  GPOut/1 -> q/1
  GPOut/3 -> vout/1
  GPIn/6 -> CB/5(nprb)
  nprb/1 -> GPIn/6

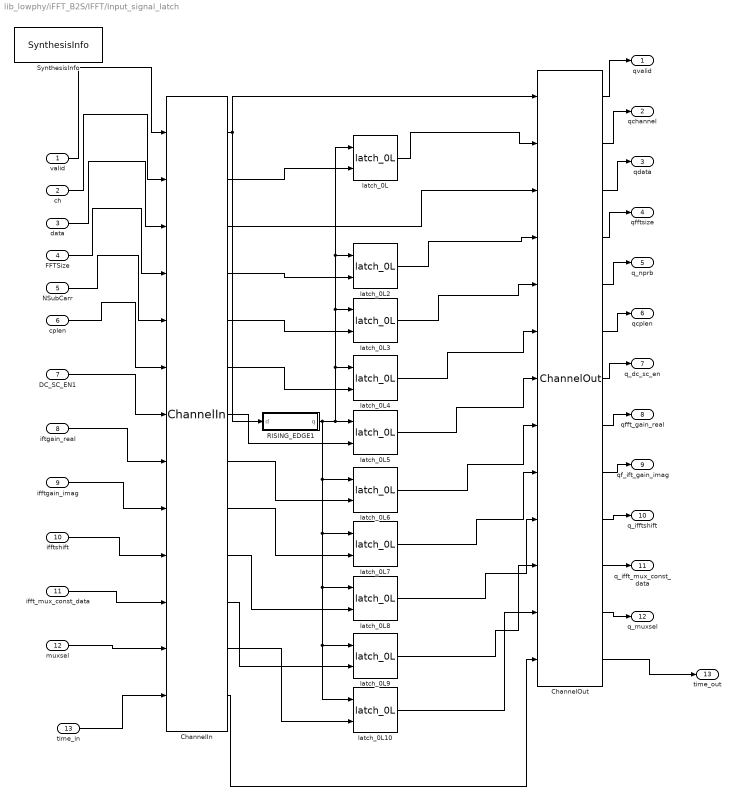
== system lib_lowphy/iFFT_B2S/IFFT/Input_signal_latch ==
  valid : Inport
  ch : Inport  Port=2
  data : Inport  Port=3
  FFTSize : Inport  Port=4
  NSubCarr : Inport  Port=5
  cplen : Inport  Port=6
  DC_SC_EN1 : Inport  Port=7
  iftgain_real : Inport  Port=8
  ifftgain_imag : Inport  Port=9
  ifftshift : Inport  Port=10
  ifft_mux_const_data : Inport  Port=11
  muxsel : Inport  Port=12
  time_in : Inport  Port=13
  ChannelIn : DSPBAPrim/ChannelIn  primtype=channelin  nInputs=dspba_internal_get_channel_ports(gcb)  nOutputs=dspba_internal_get_channel_ports(gcb)  omode=Inherit via internal rule  otype=sfix(16)  scale=2^-15  rndmethod=Unbiased  factor=1  satmethod=Symmetric  shift_vec=[0 1 2 -1]  value=11  inPortNames=['v'; 'c'; '0'; '1'; '2'; '3'; '4'; '5'; '6'; '7'; '8'; '9'; 'A'; 'B'; 'D'; 'E'; 'F'; 'G'; 'H'; 'I'; 'J'; 'K'; 'L'; 'M'; 'N'; 'O'; 'P'; 'Q'; 'R'; 'S'; 'T'; 'U'; 'W'; 'X'; 'Y'; 'Z']  outPortNames=['v'; 'c'; '0'; '1'; '2'; '3'; '4'; '5'; '6'; '7'; '8'; '9'; 'A'; 'B'; 'D'; 'E'; 'F'; 'G'; 'H'; 'I'; 'J'; 'K'; 'L'; 'M'; 'N'; 'O'; 'P'; 'Q'; 'R'; 'S'; 'T'; 'U'; 'W'; 'X'; 'Y'; 'Z']  dspbaimage=dspba_prim_channel_tall.svg  text=fprintf('In');  style=Optimised  dataSignals=11  foldingEnabled=off  channels=1  sampleRate=200  packetBeginPresent=off  packetBeginEnabled=off  visibilities=dspba_ChannelInVis(gcb)  latencyCorrection=0  scheduleOrigin=on  version=20211214
  ChannelOut : DSPBAPrim/ChannelOut  primtype=channelout  nInputs=dspba_internal_get_channel_ports(gcb)  nOutputs=dspba_internal_get_channel_ports(gcb)  omode=Inherit via internal rule  otype=sfix(16)  scale=2^-15  rndmethod=Unbiased  factor=1  satmethod=Symmetric  shift_vec=[0 1 2 -1]  value=11  inPortNames=['v'; 'c'; '0'; '1'; '2'; '3'; '4'; '5'; '6'; '7'; '8'; '9']  outPortNames=['v'; 'c'; '0'; '1'; '2'; '3'; '4'; '5'; '6'; '7'; '8'; '9']  dspbaimage=dspba_prim_channel_tall.svg  text=fprintf('Out');  style=Optimised  dataSignals=11  foldingEnabled=off  channels=1  sampleRate=200  packetBeginPresent=off  packetBeginEnabled=off  visibilities=dspba_ChannelOutVis(gcb)  latency=0  latencyCorrection=0  version=20211214
  RISING_EDGE1 : Subsystem
  SynthesisInfo : DSPBAPrim/SynthesisInfo  primtype=synthinfo  nInputs=0  nOutputs=0  omode=Inherit via internal rule  otype=sfix(16)  scale=2^-15  rndmethod=Truncate  factor=1  satmethod=Symmetric  shift_vec=[0 1 2 -1]  value=99  inPortNames=[' '; ' ';]  outPortNames=[' ']  dspbaimage=dspba_prim_ctrl.jpg  text=fprintf('Style=%s', style);  style=Scheduled  visibilities=2^17+2^18+2^19+2^20+2^21+2^22+2^23+2^24  constraintPair=None  constraintRelation=>  constraintLimit=2  modelRefSign=+  modelRef=''  showSchedule=off  simulationMode=Bit Accurate  resetMinimization=Conditional - On for ChannelIn/Out only  version=20220106
  latch_0L{,2..10} (10 alike) : DSPBAControl/latch_0L
  qvalid : Outport
  qchannel : Outport  Port=2
  qdata : Outport  Port=3
  qfftsize : Outport  Port=4
  q_nprb : Outport  Port=5
  qcplen : Outport  Port=6
  q_dc_sc_en : Outport  Port=7
  qfft_gain_real : Outport  Port=8
  qf_ift_gain_imag : Outport  Port=9
  q_ifftshift : Outport  Port=10
  q_ifft_mux_const_data : Outport  Port=11
  q_muxsel : Outport  Port=12
  time_out : Outport  Port=13
  wires:
  ChannelIn/12 -> latch_0L10/2
  valid/1 -> ChannelIn/1
  RISING_EDGE1/1(q) -> latch_0L10/1, latch_0L9/1, latch_0L8/1, latch_0L7/1, latch_0L6/1, latch_0L2/1, latch_0L/1, latch_0L3/1, latch_0L4/1, latch_0L5/1
  ChannelOut/10 -> q_ifftshift/1
  ifftgain_imag/1 -> ChannelIn/9
  ifft_mux_const_data/1 -> ChannelIn/11
  data/1 -> ChannelIn/3
  ChannelIn/2 -> latch_0L/2
  muxsel/1 -> ChannelIn/12
  ChannelIn/10 -> latch_0L8/2
  ifftshift/1 -> ChannelIn/10
  cplen/1 -> ChannelIn/6
  ChannelOut/11 -> q_ifft_mux_const_data/1
  ChannelOut/1 -> qvalid/1
  ChannelOut/2 -> qchannel/1
  ChannelIn/4 -> latch_0L2/2
  latch_0L3/1 -> ChannelOut/5
  latch_0L2/1 -> ChannelOut/4
  DC_SC_EN1/1 -> ChannelIn/7
  ChannelIn/3 -> ChannelOut/3
  latch_0L/1 -> ChannelOut/2
  ch/1 -> ChannelIn/2
  ChannelOut/9 -> qf_ift_gain_imag/1
  ChannelIn/9 -> latch_0L7/2
  latch_0L5/1 -> ChannelOut/7
  latch_0L9/1 -> ChannelOut/11
  ChannelOut/3 -> qdata/1
  ChannelOut/8 -> qfft_gain_real/1
  ChannelIn/1 -> ChannelOut/1, RISING_EDGE1/1(d)
  ChannelIn/8 -> latch_0L6/2
  NSubCarr/1 -> ChannelIn/5
  latch_0L10/1 -> ChannelOut/12
  ChannelIn/6 -> latch_0L4/2
  latch_0L8/1 -> ChannelOut/10
  ChannelIn/11 -> latch_0L9/2
  latch_0L6/1 -> ChannelOut/8
  ChannelIn/7 -> latch_0L5/2
  latch_0L4/1 -> ChannelOut/6
  ChannelOut/6 -> qcplen/1
  latch_0L7/1 -> ChannelOut/9
  iftgain_real/1 -> ChannelIn/8
  ChannelOut/5 -> q_nprb/1
  ChannelOut/4 -> qfftsize/1
  FFTSize/1 -> ChannelIn/4
  ChannelIn/5 -> latch_0L3/2
  ChannelOut/7 -> q_dc_sc_en/1
  ChannelOut/12 -> q_muxsel/1
  ChannelIn/13 -> ChannelOut/13
  time_in/1 -> ChannelIn/13
  ChannelOut/13 -> time_out/1

== system lib_lowphy/iFFT_B2S/IFFT/VIFFT ==
  data : Inport
  valid : Inport  Port=2
  channel : Inport  Port=3
  size : Inport  Port=4
  cplen : Inport  Port=5
  nsc : Inport  Port=6
  ifft_gain_re : Inport  Port=7
  ifft_gain_im : Inport  Port=8
  ifft_shift : Inport  Port=9
  ifft_mux_const : Inport  Port=10
  muxsel : Inport  Port=11
  DC_SC_EN : Inport  Port=12
  ripple_comp_en : Inport  Port=13
  rc_bw_sel : Inport  Port=14
  time_in : Inport  Port=15
  BRandSCMap : Subsystem  Opaque=on  mask(DSP Builder Advanced FFT Blockset){N=dspb_ifft_multichannel.FFTsize, subchannels=dspb_ifft_multichannel.subchannels}
      mask prompts: N "FFT Size"; subchannels "Number of subchannels (must be a power of 2)"
      mask help: Performs bit reversal of incoming FFT frames.
      mask init: same as lib_lowphy/FFT_S2B/SignalProcessing/BRandSCSelect1
      mask Help: helpview(dspba.GetHelp('BitReverseCore'));
      mask Display:
      | color('w');
      | image('dspba_fft.jpg');
      | port_label('input',1,'v');
      | port_label('input',2,'c');
      | port_label('input',3,'x');
      | port_label('input',4,'size');
      | port_label('input',5,'Nsc');
      | port_label('input',6,'cplen');
      | 
      | port_label('output',1,'qv');
      | port_label('output',2,'qc');
      | port_label('output',3,'q');
      | port_label('output',4,'ready');
      | port_label('output',6,'cp_len');
      | port_label('output',5,'size');
      | 
      | text(0.25, 0.8, 'Bit Reversal');
      | text(0.2, 0.7, 'and SubCarrier');
      | text(0.3, 0.6, 'Mapping');
      | %text(0.35,0.55,sprintf('2^{%d} to 2^{%d}',min_FFTStages, max_FFTStages),'texmode','on');
      | text(0.20,0.35,subchannelString);
  TXGainComp : Subsystem
  Terminator : Terminator
  To Workspace : ToWorkspace  Commented=on  VariableName=BR_SC_Tap_dv_out  SaveFormat=Timeseries  SampleTime=-1
  To Workspace1 : ToWorkspace  Commented=on  VariableName=BR_SC_Tap_data_out  SaveFormat=Timeseries  SampleTime=-1
  To Workspace2 : ToWorkspace  Commented=on  VariableName=iFFT_Tap_dv_out  SaveFormat=Timeseries  SampleTime=-1
  To Workspace3 : ToWorkspace  Commented=on  VariableName=iFFT_Tap_data_out  SaveFormat=Timeseries  SampleTime=-1
  To Workspace4 : ToWorkspace  Commented=on  VariableName=BR_SC_Tap_dv_in  SaveFormat=Timeseries  SampleTime=-1
  To Workspace5 : ToWorkspace  Commented=on  VariableName=BR_SC_Tap_data_in  SaveFormat=Timeseries  SampleTime=-1
  VFFT : DspbAdvFftLibrary/Common/VFFT  IFFT=dspb_ifft_multichannel.IFFT  subchannels=dspb_ifft_multichannel.subchannels  br_in=true  maxSize=dspb_ifft_multichannel.maxsize  minSize=dspb_ifft_multichannel.minsize  in_type=dspb_ifft_multichannel.InputType  type_strings=dspb_ifft_multichannel.TypeStrings  faithful=true
      link override ChannelOut1: latency=70
  dout : Outport
  vout : Outport  Port=2
  cout : Outport  Port=3
  sizeout : Outport  Port=4
  cplen_Out : Outport  Port=5
  nprb : Outport  Port=6
  fd_data_v : Outport  Port=7
  fd_data_c : Outport  Port=8
  fd_data_q : Outport  Port=9
  fd_time_out : Outport  Port=10
  wires:
  valid/1 -> To Workspace4/1, BRandSCMap/1(v)
  data/1 -> To Workspace5/1, BRandSCMap/3(x)
  TXGainComp/1(vout) -> To Workspace2/1, vout/1
  TXGainComp/3(dout) -> To Workspace3/1, dout/1
  ifft_shift/1 -> TXGainComp/8(ifft_shift)
  muxsel/1 -> TXGainComp/10(muxsel)
  VFFT/2 -> TXGainComp/2(chin)
  ifft_mux_const/1 -> TXGainComp/9(ifft_mux_const)
  BRandSCMap/6(cp_len) -> TXGainComp/5(cplen)
  VFFT/3 -> TXGainComp/4(size)
  BRandSCMap/1(qv) -> fd_data_v/1, VFFT/1, To Workspace/1  "ifft_v_in"
  BRandSCMap/5(size_out) -> VFFT/3
  channel/1 -> BRandSCMap/2(c)
  BRandSCMap/3(q) -> VFFT/4, To Workspace1/1
  BRandSCMap/2(qc) -> fd_data_c/1, VFFT/2
  ifft_gain_re/1 -> TXGainComp/6(ifft_gain_re)
  VFFT/1 -> TXGainComp/1(vin)
  size/1 -> BRandSCMap/4(FFTSize)
  nsc/1 -> nprb/1, BRandSCMap/5(NSubCarr)
  TXGainComp/5(cplen_out) -> cplen_Out/1
  ifft_gain_im/1 -> TXGainComp/7(ifft_gain_im)
  TXGainComp/4(size_out) -> sizeout/1
  VFFT/4 -> TXGainComp/3(din)
  TXGainComp/2(chout) -> cout/1
  DC_SC_EN/1 -> BRandSCMap/7(DC_SC_EN)
  BRandSCMap/4(ready) -> Terminator/1
  cplen/1 -> BRandSCMap/6(cplen)
  ripple_comp_en/1 -> BRandSCMap/8(ripple_comp_en)
  rc_bw_sel/1 -> BRandSCMap/9(rc_bw_sel)
  BRandSCMap/7(q_rc_off) -> fd_data_q/1
  time_in/1 -> BRandSCMap/10(time_in)
  BRandSCMap/8(fd_time_out) -> fd_time_out/1

== system lib_lowphy/FFT_S2B/CPRemoval/Incr_Symbol_out_val/Sym_counter_meta_data ==
  Data_write_valid : Inport
  Const3 : DSPBAPrim/Const  primtype=const  nInputs=0  nOutputs=1  omode=Inherit via internal rule  otype=sfix(16)  scale=2^-15  rndmethod=Unbiased  factor=1  satmethod=Symmetric  shift_vec=[0 1 2 -1]  value=0  inPortNames=['+'; '+';]  outPortNames=[' ']  dspbaimage=dspba_prim.svg  text=fprintf('%s', num2str(value));  style=Optimised  visibilities=8 + 1024  floatPrecision=float32_m23  warnSaturation=on  version=20211007  SampleTime=inf
  Const4 : DSPBAPrim/Const  primtype=const  nInputs=0  nOutputs=1  omode=Inherit via internal rule  otype=sfix(16)  scale=2^-15  rndmethod=Unbiased  factor=1  satmethod=Symmetric  shift_vec=[0 1 2 -1]  value=1  inPortNames=['+'; '+';]  outPortNames=[' ']  dspbaimage=dspba_prim.svg  text=fprintf('%s', num2str(value));  style=Optimised  visibilities=8 + 1024  floatPrecision=float32_m23  warnSaturation=on  version=20211007  SampleTime=inf
  Const5 : DSPBAPrim/Const  primtype=const  nInputs=0  nOutputs=1  omode=Inherit via internal rule  otype=sfix(16)  scale=2^-15  rndmethod=Unbiased  factor=1  satmethod=Symmetric  shift_vec=[0 1 2 -1]  value=14  inPortNames=['+'; '+';]  outPortNames=[' ']  dspbaimage=dspba_prim.svg  text=fprintf('%s', num2str(value));  style=Optimised  visibilities=8 + 1024  floatPrecision=float32_m23  warnSaturation=on  version=20211007  SampleTime=inf
  LoadableCounter1 : DSPBAPrim/LoadableCounter  primtype=loadablecounter  nInputs=5  nOutputs=1  omode=Specify via dialog  otype=ufix(4)  scale=2^-0  rndmethod=Unbiased  factor=1  satmethod=Symmetric  shift_vec=[0 1 2 -1]  value=[0 14 1]  inPortNames=['en';'ld';'i ';'s ';'m ']  outPortNames=[' ']  dspbaimage=dspba_prim_tall.svg  text=fprintf('loadable\ncounter\n[%d %d %d]', value(1), value(2), value(3));  style=Optimised  visibilities=8 + 1024  version=20211007
  Rising edge1 : Subsystem
  SampleDelay3 : DSPBAPrim/SampleDelay  primtype=sampdelay  nInputs=1  nOutputs=1  omode=Inherit via internal rule  otype=sfix(16)  scale=2^-15  rndmethod=Unbiased  factor=1  satmethod=Symmetric  shift_vec=[0 1 2 -1]  floatPrecision=float32_m23  value=1  inPortNames=[' '; ' ';]  outPortNames=[' ']  dspbaimage=dspba_prim.svg  text=dpoly(1, eye(1,value+1), 'z')  style=Optimised  visibilities=8 + 1024 + 2^17 + 2^18  flexible=off  slackgroup=0  augmented=0  version=20211007  advOptions=[]
  Subsystem : Subsystem
  Sym_out_meta : Outport
  wires:
  Const3/1 -> LoadableCounter1/3
  Const5/1 -> LoadableCounter1/5
  Rising edge1/1(q) -> LoadableCounter1/1
  LoadableCounter1/1 -> Sym_out_meta/1, Subsystem/1(cntr)
  Subsystem/1(sym1_det) -> SampleDelay3/1
  Const4/1 -> LoadableCounter1/4
  SampleDelay3/1 -> LoadableCounter1/2
  Data_write_valid/1 -> Rising edge1/1(d)

== system lib_lowphy/FFT_S2B/CPRemoval/Mem_rd_sub1/Incr_Symbol_out_val ==
  dv : Inport
  Sym_counter_meta_data : Subsystem
  Sym_out_meta : Outport
  wires:
  Sym_counter_meta_data/1(Sym_out_meta) -> Sym_out_meta/1
  dv/1 -> Sym_counter_meta_data/1(Data_write_valid)
